simulink model "PEMEC_smlk"  (R2015b)
settings: Solver=VariableStepAuto  SolverMode=SingleTasking  StartTime=0.0  StopTime=1000  MaxStep=1  MinStep=0.0001  RelTol=1e-3
values from neighbouring files (symbols this model uses):
  a = 1 / tau_th + C_cw / C_th * (1 - exp(-UA / C_cw))    [PEMEC_cellstack.m]    (also in PEMEC_data.m = 0.000364)
  A_cell = 0.0170    (= 0.017)    [PEMEC_begin.m]
  alpha_an = 2    [PEMEC_cellstack.m]    (also in PEMEC_data.m)
  alpha_cat = 0.5    [PEMEC_cellstack.m]    (also in PEMEC_data.m)
  b = N_cell * V_ * I * (1 - eta_e) / C_th + T_amb / tau_th +      C_cw * T_cwin / C_th * (1 - exp(-UA / C_cw))    [PEMEC_cellstack.m]    (also in PEMEC_data.m = 2.334)
  C = 0.008    [PEMEC_data.m]
  c_cw = 4.18e03    (= 4180)    [PEMEC_cellstack.m]    (also in PEMEC_data.m)
  C_th = 250e03    (= 250000)    [PEMEC_data.m]
  cH2_me0 = 10.0    (= 10)    [PEMEC_data.m]
  cO2_me0 = 0.10    (= 0.1)    [PEMEC_data.m]
  Deff_an0 = Deff_an_  * 1e04    [PEMEC_data.m]
  Deff_cat0 = Deff_cat_ * 1e04    [PEMEC_data.m]
  DeltaP = (p_an - p_atm) / eta_p    [PEMEC_data.m]
  Dw = 1.28e-10    [PEMEC_cellstack.m]    (also in PEMEC_data.m)
  Epro = 20000    [PEMEC_data.m]
  eta_ACDC = 0.96    [PEMEC_data.m]
  F = 96485    [PEMEC_begin.m]
  f1 = 25000    [PEMEC_data.m]
  f2 = 0.98    [PEMEC_data.m]
  h_cond = 380    [PEMEC_data.m]
  h_conv = 0.1    [PEMEC_data.m]
  K2 = 1 / (2 * A * io_an)    [PEMEC_cellstack.m]    (also in PEMEC_data.m = 1 / (2 * A_cell * io_an))
  K4 = 1 / (2 * A * io_cat)    [PEMEC_cellstack.m]    (also in PEMEC_data.m = 1 / (2 * A_cell * io_cat))
  K_H2 = n_H2r / p_H2out    [PEMEC_data.m]
  K_H2O = n_H2Oout / p_H2Oout    [PEMEC_data.m]
  K_O2 = n_O2r / p_O2out    [PEMEC_data.m]
  K_r = N_cell / (4 * F)    [PEMEC_data.m]
  m_cw = 0.1075    [PEMEC_cellstack.m]    (also in PEMEC_data.m = 0.25)
  M_H2 = 2.01588    [PEMEC_cellstack.m]    (also in PEMEC_data.m)
  M_H2O = 18.01528    [PEMEC_cellstack.m]    (also in PEMEC_data.m)
  M_O2 = 31.9988    [PEMEC_cellstack.m]    (also in PEMEC_data.m)
  N_cell = 200    [PEMEC_begin.m]
  n_H2Omem2 = 1 - Dw / t_mem * (t_cat / Deff_cat + t_an / Deff_an)    [PEMEC_cellstack.m]    (also in PEMEC_data.m = 1 - Dw / t_mem * (t_cat / Deff_cat_ + t_an / Deff_an_))
  n_H2Opg = Kw * A * rho_H2O / (mu_H2O * M_H2O * t_mem) * (p_cat - p_an)    [PEMEC_cellstack.m]    (also in PEMEC_data.m = Kw * A_cell * rho_H2O / (mu_H2O * M_H2O * t_mem)*(p_cat - p_)
  nd = 7    [PEMEC_cellstack.m]    (also in PEMEC_data.m)
  p_an = p_atm * 50    (= 5066250)    [PEMEC_begin.m]
  p_cat = p_atm * 50    (= 5066250)    [PEMEC_begin.m]
  P_gamma = 2.5e03    (= 2500)    [PEMEC_data.m]
  p_H20 = y_H2O * p_an / 101325    [PEMEC_data.m]
  p_H2O0 = y_H2 * p_an / 101325    [PEMEC_data.m]
  p_O20 = y_O2 * p_cat / 101325    [PEMEC_data.m]
  R = 8.314    [PEMEC_begin.m]
  R_th = 0.0817    [PEMEC_data.m]
  Req_el = 180e-06    (= 0.00018)    [PEMEC_data.m]
  rho_H2O = 1000    [PEMEC_cellstack.m]    (also in PEMEC_data.m = 999.7)
  T = 80 + 273.15    (= 353.15)    [PEMEC_begin.m]
  T0 = T_a    [PEMEC_data.m]
  T_a = 25    [PEMEC_begin.m]
  T_amb = 25    [PEMEC_begin.m]    (also in PEMEC_data.m = T_a + 273.15)
  t_an = 0.00020    (= 0.0002)    [PEMEC_data.m]
  t_cat = 0.00020    (= 0.0002)    [PEMEC_data.m]
  T_cwin = 20 + 0    (= 20)    [PEMEC_cellstack.m]    (also in PEMEC_data.m)
  T_des = T - 273.15    [PEMEC_data.m]
  t_mem = 0.00020    (= 0.0002)    [PEMEC_data.m]
  T_ref = 327.15    [PEMEC_begin.m]
  tau_H2 = 2.07    [PEMEC_data.m]
  tau_O2 = 4.14    [PEMEC_data.m]
  tau_p = 0.5    [PEMEC_data.m]
  tau_th = C_th * R_th    [PEMEC_cellstack.m]    (also in PEMEC_data.m = 20425)
  U = polyval(polU, I(1))    [PEMEC_data.m]
  v_H240 = 3.1777e03    (= 3177.7)    [PEMEC_data.m]
  v_H2O = 999.97e03    (= 999970)    [PEMEC_cellstack.m]    (also in PEMEC_data.m = 999700)
  v_O240 = 52.876e03    (= 52876)    [PEMEC_data.m]
  V_tn = 1.48    [PEMEC_cellstack.m]    (also in PEMEC_data.m)
  VS_H2 = 40    [PEMEC_data.m]
  VS_O2 = 20    [PEMEC_data.m]
  y_H2 = 0.005    [PEMEC_begin.m]
  y_O2 = 0.005    [PEMEC_begin.m]
  zeta = 1    [PEMEC_data.m]
undefined symbols (not defined in the file or in its folder): magnitude
settings Model: Creator=gapaolo  LastModifiedBy=gapaolo
settings DataIOCC: SaveFormat=Array
settings OptimizationCC: BlockReduction=off  BooleanDataType=off
settings DebuggingCC: AlgebraicLoopMsg=none  SaveWithParameterizedLinksMsg=none  UnderspecifiedInitializationDetection=Classic  MergeDetectMultiDrivingBlocksExec=none  SignalResolutionControl=TryResolveAllWithWarning
settings HardwareCC: ProdBitPerPointer=32  ProdLargestAtomicFloat=None  ProdIntDivRoundTo=Undefined  ProdEndianess=Unspecified  ProdWordSize=32  ProdHWDeviceType=32-bit Generic  TargetUnknown=on
settings GRTTargetCC: GeneratePreprocessorConditionals=Disable all
settings ConfigComp: CovModelRefEnable=Off  CovSFcnEnable=off

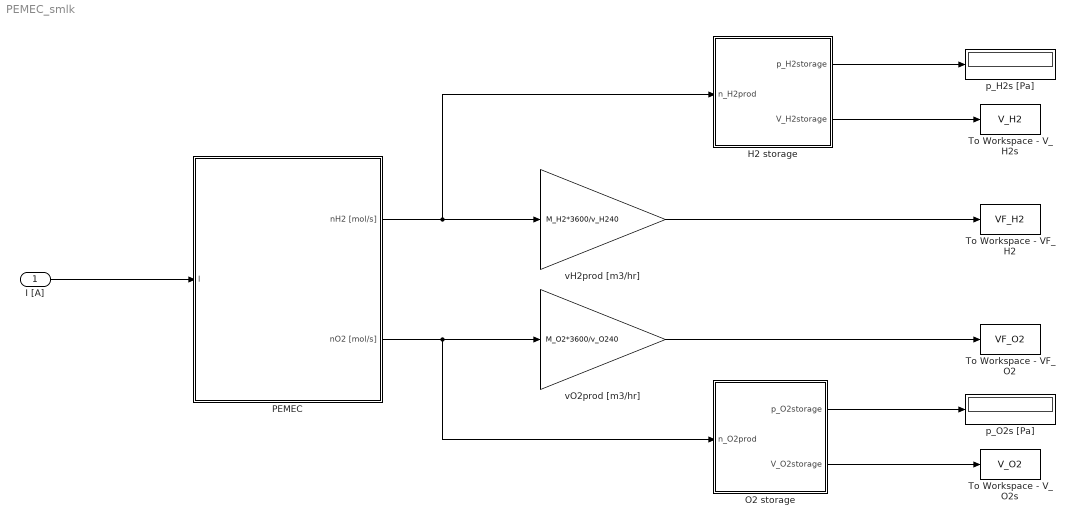
== system PEMEC_smlk ==
  I [A] : Inport
  H2 storage : Subsystem
  O2 storage : Subsystem
  PEMEC : Subsystem
  To Workspace - VF_H2 : ToWorkspace  VariableName=VF_H2  SaveFormat=Timeseries  SampleTime=-1
  To Workspace - VF_O2 : ToWorkspace  VariableName=VF_O2  SaveFormat=Timeseries  SampleTime=-1
  To Workspace - V_H2s : ToWorkspace  VariableName=V_H2  SaveFormat=Timeseries  SampleTime=-1
  To Workspace - V_O2s : ToWorkspace  VariableName=V_O2  SaveFormat=Timeseries  SampleTime=-1
  p_H2s [Pa] : Display
  p_O2s [Pa] : Display
  vH2prod [m3/hr] : Gain  Gain=M_H2*3600/v_H240
  vO2prod [m3/hr] : Gain  Gain=M_O2*3600/v_O240
  wires:
  I [A]/1 -> PEMEC/1(I)
  H2 storage/1(p_H2storage) -> p_H2s [Pa]/1
  PEMEC/2(nO2 [mol/s]) -> O2 storage/1(n_O2prod), vO2prod [m3/hr]/1
  O2 storage/1(p_O2storage) -> p_O2s [Pa]/1
  H2 storage/2(V_H2storage) -> To Workspace - V_H2s/1
  O2 storage/2(V_O2storage) -> To Workspace - V_O2s/1
  vH2prod [m3/hr]/1 -> To Workspace - VF_H2/1
  vO2prod [m3/hr]/1 -> To Workspace - VF_O2/1
  PEMEC/1(nH2 [mol/s]) -> H2 storage/1(n_H2prod), vH2prod [m3/hr]/1

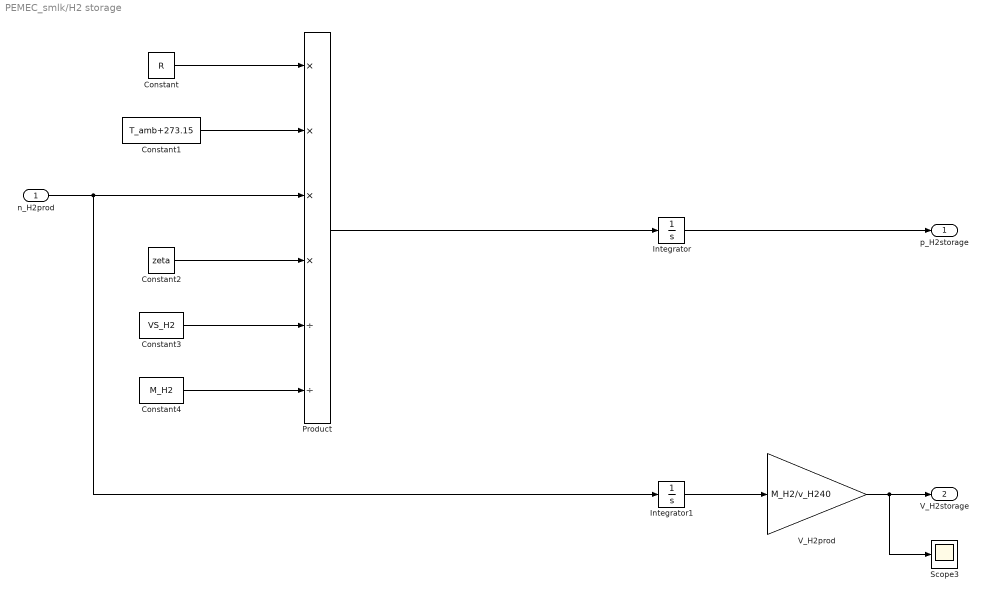
== system PEMEC_smlk/H2 storage ==
  n_H2prod : Inport
  Constant : Constant  Value=R
  Constant1 : Constant  Value=T_amb+273.15
  Constant2 : Constant  Value=zeta
  Constant3 : Constant  Value=VS_H2
  Constant4 : Constant  Value=M_H2
  Integrator : Integrator  InitialCondition=101325
  Integrator1 : Integrator
  Product : Product  Inputs=****//
  Scope3 : Scope
  V_H2prod : Gain  Gain=M_H2/v_H240
  p_H2storage : Outport
  V_H2storage : Outport  Port=2
  wires:
  n_H2prod/1 -> Integrator1/1, Product/3
  Constant/1 -> Product/1
  Constant1/1 -> Product/2
  Constant2/1 -> Product/4
  Constant3/1 -> Product/5
  Constant4/1 -> Product/6
  Product/1 -> Integrator/1
  Integrator/1 -> p_H2storage/1
  Integrator1/1 -> V_H2prod/1
  V_H2prod/1 -> Scope3/1, V_H2storage/1

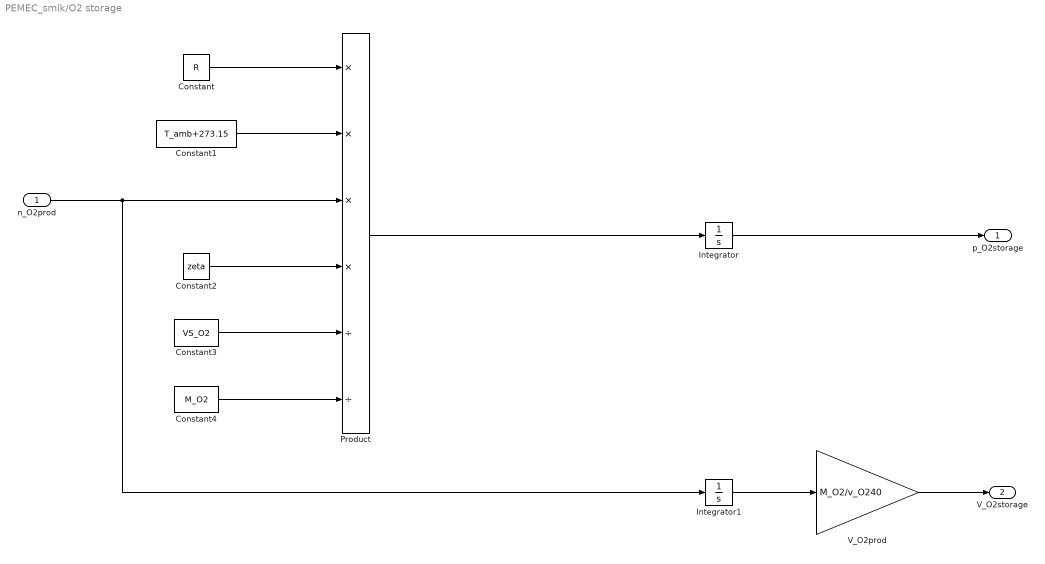
== system PEMEC_smlk/O2 storage ==
  n_O2prod : Inport
  Constant : Constant  Value=R
  Constant1 : Constant  Value=T_amb+273.15
  Constant2 : Constant  Value=zeta
  Constant3 : Constant  Value=VS_O2
  Constant4 : Constant  Value=M_O2
  Integrator : Integrator  InitialCondition=101325
  Integrator1 : Integrator
  Product : Product  Inputs=****//
  V_O2prod : Gain  Gain=M_O2/v_O240
  p_O2storage : Outport
  V_O2storage : Outport  Port=2
  wires:
  n_O2prod/1 -> Integrator1/1, Product/3
  Constant/1 -> Product/1
  Constant1/1 -> Product/2
  Constant2/1 -> Product/4
  Constant3/1 -> Product/5
  Constant4/1 -> Product/6
  Product/1 -> Integrator/1
  Integrator/1 -> p_O2storage/1
  Integrator1/1 -> V_O2prod/1
  V_O2prod/1 -> V_O2storage/1

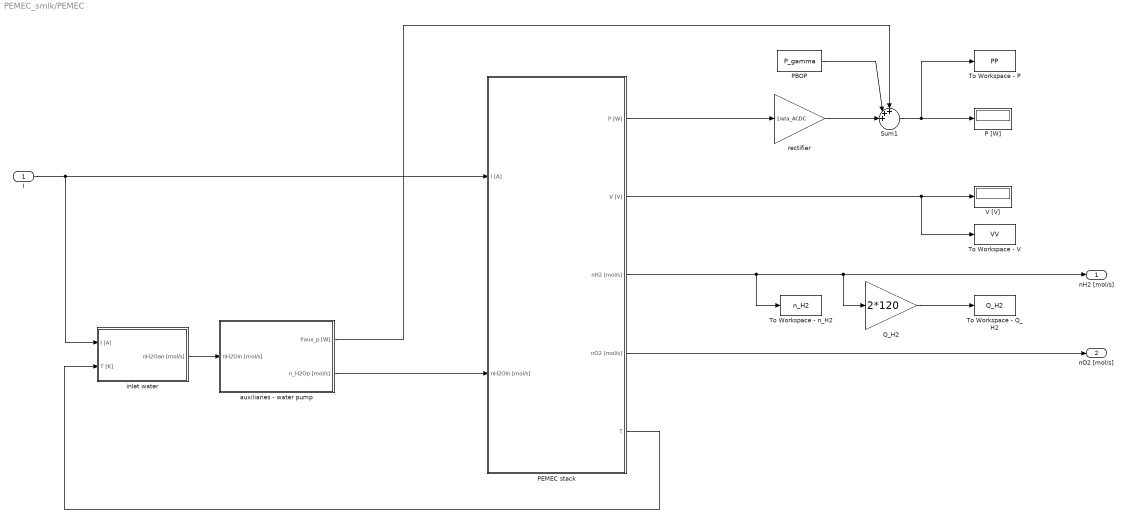
== system PEMEC_smlk/PEMEC ==
  I : Inport
  P [W] : Display
  PBOP : Constant  Value=P_gamma
  PEMEC stack : Subsystem
  Q_H2 : Gain  Gain=2*120
  Sum1 : Sum  Inputs=+++||
  To Workspace - P : ToWorkspace  VariableName=PP  SaveFormat=Timeseries  SampleTime=-1
  To Workspace - Q_H2 : ToWorkspace  VariableName=Q_H2  SaveFormat=Timeseries  SampleTime=-1
  To Workspace - V : ToWorkspace  VariableName=VV  SaveFormat=Timeseries  SampleTime=-1
  To Workspace - n_H2 : ToWorkspace  VariableName=n_H2  SaveFormat=Timeseries  SampleTime=-1
  V [V] : Display
  auxiliaries - water pump : Subsystem
  inlet water : Subsystem
  rectifier : Gain  Gain=1/eta_ACDC
  nH2 [mol/s] : Outport
  nO2 [mol/s] : Outport  Port=2
  wires:
  PEMEC stack/2(V [V]) -> To Workspace - V/1, V [V]/1
  I/1 -> inlet water/1(I [A]), PEMEC stack/1(I [A])
  PEMEC stack/1(P [W]) -> rectifier/1
  inlet water/1("nH2Oan [mol/s] ") -> auxiliaries - water pump/1(nH2Oin [mol/s])
  auxiliaries - water pump/2(n_H2Op [mol/s]) -> PEMEC stack/2(nH2Oin [mol/s])
  rectifier/1 -> Sum1/3
  Sum1/1 -> To Workspace - P/1, P [W]/1
  PBOP/1 -> Sum1/2
  auxiliaries - water pump/1(Paux_p [W]) -> Sum1/1
  PEMEC stack/5(T) -> inlet water/2(T [K])
  PEMEC stack/4(nO2 [mol/s]) -> nO2 [mol/s]/1
  PEMEC stack/3(nH2 [mol/s]) -> Q_H2/1, nH2 [mol/s]/1, To Workspace - n_H2/1
  Q_H2/1 -> To Workspace - Q_H2/1

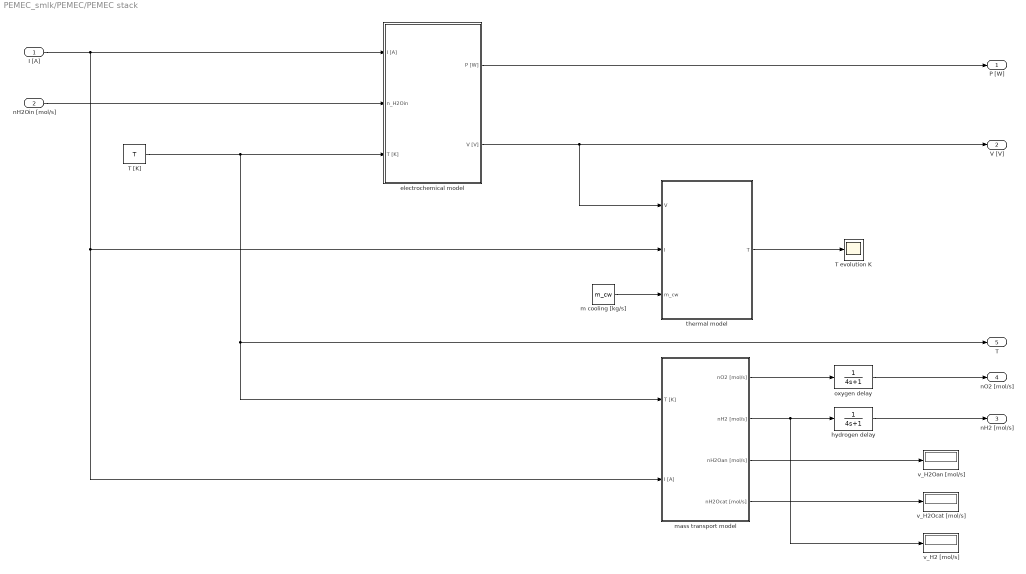
== system PEMEC_smlk/PEMEC/PEMEC stack ==
  I [A] : Inport
  nH2Oin [mol/s] : Inport  Port=2
  T [K] : Constant  Value=T
  T evolution K : Scope
  electrochemical model : Subsystem
  hydrogen delay : TransferFcn  Denominator=[4 1]
  m cooling [kg/s] : Constant  Value=m_cw
  mass transport model : Subsystem
  oxygen delay : TransferFcn  Denominator=[4 1]
  thermal model : Subsystem
  v_H2 [mol/s] : Display
  v_H2Oan [mol/s] : Display
  v_H2Ocat [mol/s] : Display
  P [W] : Outport
  V [V] : Outport  Port=2
  nH2 [mol/s] : Outport  Port=3
  nO2 [mol/s] : Outport  Port=4
  T : Outport  Port=5
  wires:
  m cooling [kg/s]/1 -> thermal model/3(m_cw)
  electrochemical model/2(V [V]) -> V [V]/1, thermal model/1(V)
  thermal model/1(T) -> T evolution K/1
  electrochemical model/1(P [W]) -> P [W]/1
  I [A]/1 -> thermal model/2(I), mass transport model/2(I [A]), electrochemical model/1(I [A])
  nH2Oin [mol/s]/1 -> electrochemical model/2(n_H2Oin)
  T [K]/1 -> T/1, mass transport model/1(T [K]), electrochemical model/3(T [K])
  oxygen delay/1 -> nO2 [mol/s]/1
  hydrogen delay/1 -> nH2 [mol/s]/1
  mass transport model/1(nO2 [mol/s]) -> oxygen delay/1
  mass transport model/2(nH2 [mol/s]) -> v_H2 [mol/s]/1, hydrogen delay/1
  mass transport model/3(nH2Oan [mol/s]) -> v_H2Oan [mol/s]/1
  mass transport model/4(nH2Ocat [mol/s]) -> v_H2Ocat [mol/s]/1

== system PEMEC_smlk/PEMEC/auxiliaries - water pump ==
  nH2Oin [mol/s] : Inport
  Display : Display
  Paux pump : Gain  Gain=DeltaP
  nH2Oin : Gain  Gain=rho_H2O/M_H2O
  pump delay : TransferFcn  Denominator=[tau_p 1]
  vH2in [m3/s] : Gain  Gain=M_H2O/v_H2O
  vH2in [m3/s]1 : Gain  Gain=M_H2O
  Paux_p [W] : Outport
  n_H2Op [mol/s] : Outport  Port=2
  wires:
  vH2in [m3/s]/1 -> pump delay/1
  nH2Oin/1 -> n_H2Op [mol/s]/1
  Paux pump/1 -> Paux_p [W]/1
  nH2Oin [mol/s]/1 -> vH2in [m3/s]1/1, vH2in [m3/s]/1
  pump delay/1 -> nH2Oin/1, Paux pump/1
  vH2in [m3/s]1/1 -> Display/1

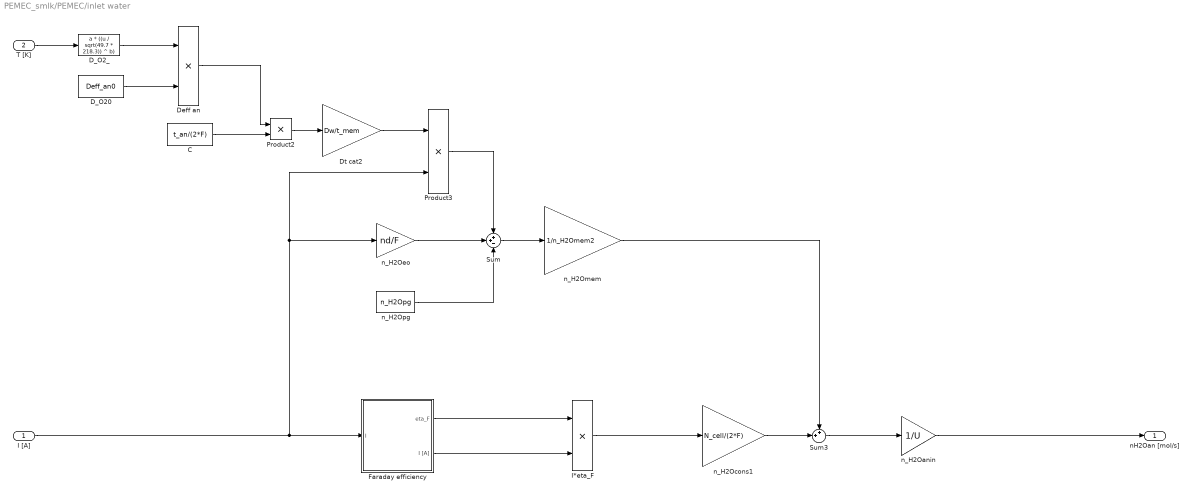
== system PEMEC_smlk/PEMEC/inlet water ==
  I [A] : Inport
  T [K] : Inport  Port=2
  C : Constant  Value=t_an/(2*F)
  D_O20 : Constant  Value=Deff_an0
  D_O2_ : Fcn  Expr=a * ((u / sqrt(49.7 * 218.3)) ^ b)
  Deff an : Product
  Dt cat2 : Gain  Gain=Dw/t_mem
  Faraday efficiency : Subsystem
  I*eta_F : Product
  Product2 : Product
  Product3 : Product
  Sum : Sum  Inputs=++-
  Sum3 : Sum  Inputs=++|
  n_H2Oanin : Gain  Gain=1/U
  n_H2Ocons1 : Gain  Gain=N_cell/(2*F)
  n_H2Oeo : Gain  Gain=nd/F
  n_H2Omem : Gain  Gain=1/n_H2Omem2
  n_H2Opg : Constant  Value=n_H2Opg
  "nH2Oan [mol/s] " : Outport
  wires:
  Faraday efficiency/2(I [A]) -> I*eta_F/2
  Faraday efficiency/1(eta_F) -> I*eta_F/1
  I*eta_F/1 -> n_H2Ocons1/1
  n_H2Opg/1 -> Sum/3
  n_H2Oeo/1 -> Sum/2
  n_H2Ocons1/1 -> Sum3/2
  Sum3/1 -> n_H2Oanin/1
  n_H2Oanin/1 -> "nH2Oan [mol/s] "/1
  Sum/1 -> n_H2Omem/1
  n_H2Omem/1 -> Sum3/1
  I [A]/1 -> Product3/2, n_H2Oeo/1, Faraday efficiency/1(I)
  T [K]/1 -> D_O2_/1
  D_O2_/1 -> Deff an/1
  D_O20/1 -> Deff an/2
  Deff an/1 -> Product2/1
  C/1 -> Product2/2
  Product2/1 -> Dt cat2/1
  Dt cat2/1 -> Product3/1
  Product3/1 -> Sum/1

== system PEMEC_smlk/PEMEC/PEMEC stack/electrochemical model ==
  I [A] : Inport
  n_H2Oin : Inport  Port=2
  T [K] : Inport  Port=3
  Nernst voltage : Subsystem
  P : Product
  "voltage losses " : Subsystem
  P [W] : Outport
  V [V] : Outport  Port=2
  wires:
  I [A]/1 -> Nernst voltage/2(I [A]), "voltage losses "/1(I [A])
  "voltage losses "/1(V) -> P/1, V [V]/1
  P/1 -> P [W]/1
  T [K]/1 -> Nernst voltage/1(T [K]), "voltage losses "/2(T [K])
  "voltage losses "/2(I) -> P/2
  n_H2Oin/1 -> Nernst voltage/3(n_H2Oin)
  Nernst voltage/1(E) -> "voltage losses "/3(E [V])

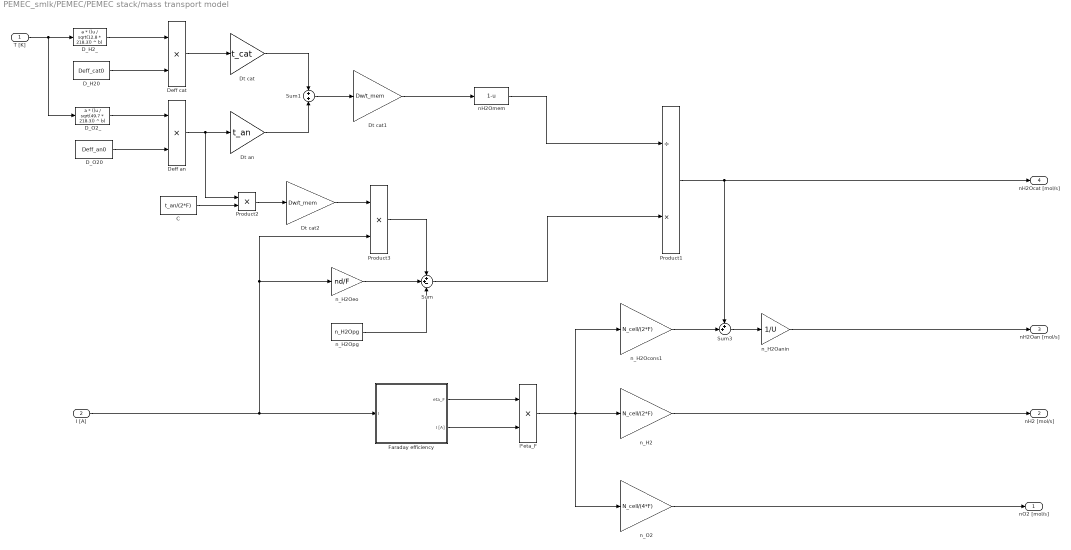
== system PEMEC_smlk/PEMEC/PEMEC stack/mass transport model ==
  T [K] : Inport
  I [A] : Inport  Port=2
  C : Constant  Value=t_an/(2*F)
  D_H20 : Constant  Value=Deff_cat0
  D_H2_ : Fcn  Expr=a * ((u / sqrt(12.8 * 218.3)) ^ b)
  D_O20 : Constant  Value=Deff_an0
  D_O2_ : Fcn  Expr=a * ((u / sqrt(49.7 * 218.3)) ^ b)
  Deff an : Product
  Deff cat : Product
  Dt an : Gain  Gain=t_an
  Dt cat : Gain  Gain=t_cat
  Dt cat1 : Gain  Gain=Dw/t_mem
  Dt cat2 : Gain  Gain=Dw/t_mem
  Faraday efficiency : Subsystem
  I*eta_F : Product
  Product1 : Product  Inputs=/*
  Product2 : Product
  Product3 : Product
  Sum : Sum  Inputs=++-
  Sum1 : Sum  Inputs=+|+
  Sum3 : Sum  Inputs=++|
  nH2Omem : Fcn  Expr=1-u
  n_H2 : Gain  Gain=N_cell/(2*F)
  n_H2Oanin : Gain  Gain=1/U
  n_H2Ocons1 : Gain  Gain=N_cell/(2*F)
  n_H2Oeo : Gain  Gain=nd/F
  n_H2Opg : Constant  Value=n_H2Opg
  n_O2 : Gain  Gain=N_cell/(4*F)
  nO2 [mol/s] : Outport
  nH2 [mol/s] : Outport  Port=2
  nH2Oan [mol/s] : Outport  Port=3
  nH2Ocat [mol/s] : Outport  Port=4
  wires:
  Faraday efficiency/2(I [A]) -> I*eta_F/2
  Faraday efficiency/1(eta_F) -> I*eta_F/1
  n_H2/1 -> nH2 [mol/s]/1
  n_O2/1 -> nO2 [mol/s]/1
  I [A]/1 -> Faraday efficiency/1(I), Product3/2, n_H2Oeo/1
  I*eta_F/1 -> n_H2Ocons1/1, n_H2/1, n_O2/1
  n_H2Opg/1 -> Sum/3
  n_H2Oeo/1 -> Sum/2
  n_H2Ocons1/1 -> Sum3/2
  Sum3/1 -> n_H2Oanin/1
  n_H2Oanin/1 -> nH2Oan [mol/s]/1
  T [K]/1 -> D_H2_/1, D_O2_/1
  D_H2_/1 -> Deff cat/1
  D_O2_/1 -> Deff an/1
  D_H20/1 -> Deff cat/2
  D_O20/1 -> Deff an/2
  Deff cat/1 -> Dt cat/1
  Deff an/1 -> Product2/1, Dt an/1
  Dt cat/1 -> Sum1/1
  Dt an/1 -> Sum1/2
  Sum1/1 -> Dt cat1/1
  Dt cat1/1 -> nH2Omem/1
  Sum/1 -> Product1/2
  nH2Omem/1 -> Product1/1
  Product1/1 -> Sum3/1, nH2Ocat [mol/s]/1
  C/1 -> Product2/2
  Product2/1 -> Dt cat2/1
  Dt cat2/1 -> Product3/1
  Product3/1 -> Sum/1

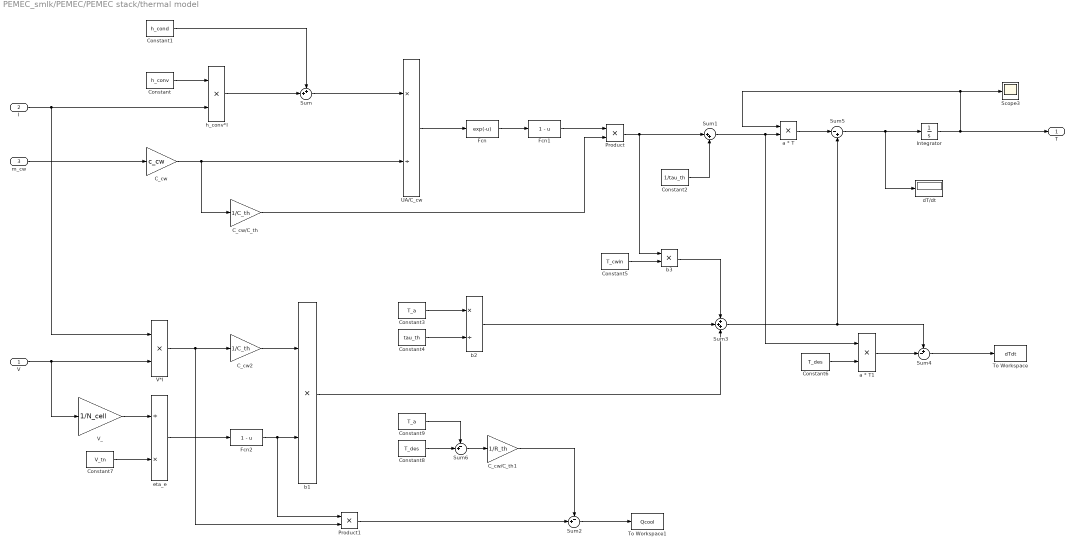
== system PEMEC_smlk/PEMEC/PEMEC stack/thermal model ==
  V : Inport
  I : Inport  Port=2
  m_cw : Inport  Port=3
  C_cw : Gain  Gain=c_cw
  C_cw/C_th : Gain  Gain=1/C_th
  C_cw/C_th1 : Gain  Gain=1/R_th
  C_cw2 : Gain  Gain=1/C_th
  Constant : Constant  Value=h_conv
  Constant1 : Constant  Value=h_cond
  Constant2 : Constant  Value=1/tau_th
  Constant3 : Constant  Value=T_a
  Constant4 : Constant  Value=tau_th
  Constant5 : Constant  Value=T_cwin
  Constant6 : Constant  Value=T_des
  Constant7 : Constant  Value=V_tn
  Constant8 : Constant  Value=T_des
  Constant9 : Constant  Value=T_a
  Fcn : Fcn  Expr=exp(-u)
  Fcn1 : Fcn  Expr=1 - u
  Fcn2 : Fcn  Expr=1 - u
  Integrator : Integrator  InitialCondition=T0
  Product : Product
  Product1 : Product
  Scope3 : Scope
  Sum : Sum  Inputs=++|
  Sum1 : Sum  Inputs=|++
  Sum2 : Sum  Inputs=-+|
  Sum3 : Sum  Inputs=+++
  Sum4 : Sum  Inputs=+-|
  Sum5 : Sum  Inputs=|-+
  Sum6 : Sum  Inputs=-+|
  To Workspace : ToWorkspace  VariableName=dTdt  SaveFormat=Timeseries  SampleTime=-1
  To Workspace1 : ToWorkspace  VariableName=Qcool  SaveFormat=Timeseries  SampleTime=-1
  UA/C_cw : Product  Inputs=*/
  V*I : Product
  V_ : Gain  Gain=1/N_cell
  a * T : Product
  a * T1 : Product
  b1 : Product
  b2 : Product  Inputs=*/
  b3 : Product
  dT/dt : Display
  eta_e : Product  Inputs=/*
  h_conv*I : Product
  T : Outport
  wires:
  I/1 -> V*I/1, h_conv*I/2
  Constant/1 -> h_conv*I/1
  h_conv*I/1 -> Sum/2
  Constant1/1 -> Sum/1
  Sum/1 -> UA/C_cw/1
  m_cw/1 -> C_cw/1
  UA/C_cw/1 -> Fcn/1
  Fcn/1 -> Fcn1/1
  C_cw/1 -> UA/C_cw/2, C_cw/C_th/1
  Fcn1/1 -> Product/1
  C_cw/C_th/1 -> Product/2
  Product/1 -> b3/1, Sum1/1
  Constant2/1 -> Sum1/2
  C_cw2/1 -> b1/1
  Constant3/1 -> b2/1
  Constant4/1 -> b2/2
  Constant5/1 -> b3/2
  b3/1 -> Sum3/1
  b2/1 -> Sum3/2
  V_/1 -> eta_e/1
  Constant7/1 -> eta_e/2
  eta_e/1 -> Fcn2/1
  Sum5/1 -> dT/dt/1, Integrator/1
  a * T/1 -> Sum5/1
  Sum1/1 -> a * T1/1, a * T/2
  Integrator/1 -> a * T/1, Scope3/1, T/1
  b1/1 -> Sum3/3
  Sum3/1 -> Sum4/1, Sum5/2
  Constant6/1 -> a * T1/2
  Sum4/1 -> To Workspace/1
  a * T1/1 -> Sum4/2
  Product1/1 -> Sum2/2
  Constant8/1 -> Sum6/2
  Constant9/1 -> Sum6/1
  Sum6/1 -> C_cw/C_th1/1
  C_cw/C_th1/1 -> Sum2/1
  Sum2/1 -> To Workspace1/1
  V*I/1 -> Product1/2, C_cw2/1
  Fcn2/1 -> Product1/1, b1/2
  V/1 -> V*I/2, V_/1

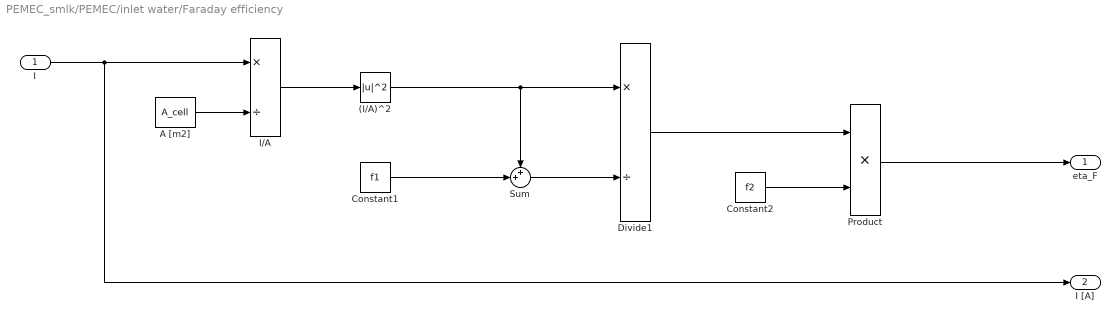
== system PEMEC_smlk/PEMEC/inlet water/Faraday efficiency ==
  I : Inport
  (I/A)^2 : Math  Operator=magnitude^2  SaturateOnIntegerOverflow=on
  A [m2] : Constant  Value=A_cell
  Constant1 : Constant  Value=f1
  Constant2 : Constant  Value=f2
  Divide1 : Product  Inputs=*/
  I/A : Product  Inputs=*/
  Product : Product
  Sum : Sum  Inputs=++|
  eta_F : Outport
  I [A] : Outport  Port=2
  wires:
  A [m2]/1 -> I/A/2
  I/1 -> I [A]/1, I/A/1
  I/A/1 -> (I/A)^2/1
  (I/A)^2/1 -> Sum/1, Divide1/1
  Constant1/1 -> Sum/2
  Sum/1 -> Divide1/2
  Divide1/1 -> Product/1
  Constant2/1 -> Product/2
  Product/1 -> eta_F/1

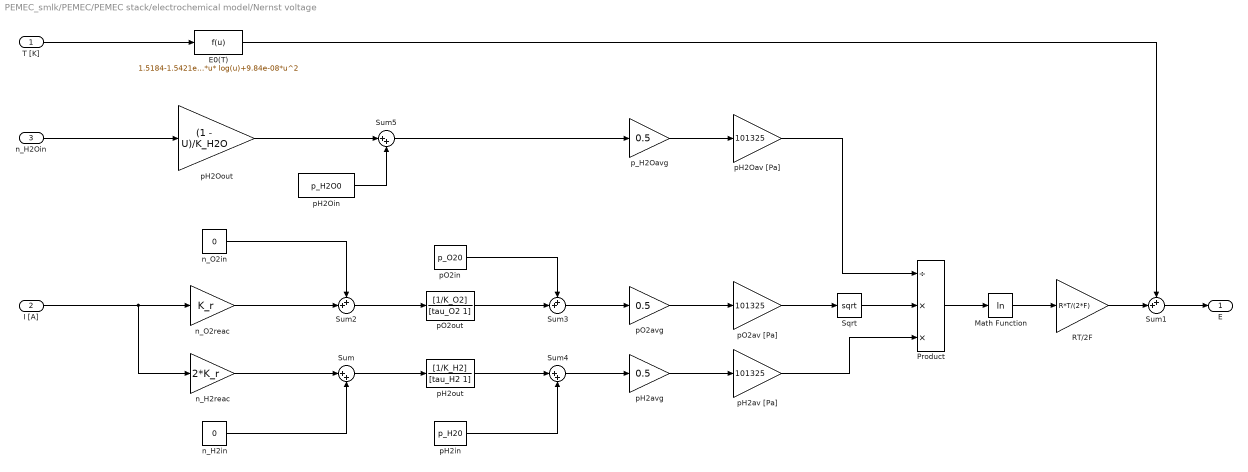
== system PEMEC_smlk/PEMEC/PEMEC stack/electrochemical model/Nernst voltage ==
  T [K] : Inport
  I [A] : Inport  Port=2
  n_H2Oin : Inport  Port=3
  E0(T) : Fcn  Expr=1.5184-1.5421e-03*u+9.523e-05*u* log(u)+9.84e-08*u^2
  Math Function : Math  Operator=log  SaturateOnIntegerOverflow=on
  Product : Product  Inputs=/**
  RT/2F : Gain  Gain=R*T/(2*F)
  Sqrt : Sqrt  SaturateOnIntegerOverflow=on
  Sum : Sum  Inputs=|++
  Sum1 : Sum  Inputs=++|
  Sum2 : Sum  Inputs=++|
  Sum3 : Sum  Inputs=++|
  Sum4 : Sum  Inputs=|++
  Sum5 : Sum  Inputs=|++
  n_H2in : Constant  Value=0
  n_H2reac : Gain  Gain=2*K_r
  n_O2in : Constant  Value=0
  n_O2reac : Gain  Gain=K_r
  pH2Oav [Pa] : Gain  Gain=101325
  pH2Oin : Constant  Value=p_H2O0
  pH2Oout : Gain  Gain=(1 - U)/K_H2O
  pH2av [Pa] : Gain  Gain=101325
  pH2avg : Gain  Gain=0.5
  pH2in : Constant  Value=p_H20
  pH2out : TransferFcn  Numerator=[1/K_H2]  Denominator=[tau_H2 1]  ContinuousStateAttributes='p_H2'
  pO2av [Pa] : Gain  Gain=101325
  pO2avg : Gain  Gain=0.5
  pO2in : Constant  Value=p_O20
  pO2out : TransferFcn  Numerator=[1/K_O2]  Denominator=[tau_O2 1]  ContinuousStateAttributes='p_O2'
  p_H2Oavg : Gain  Gain=0.5
  E : Outport
  wires:
  I [A]/1 -> n_O2reac/1, n_H2reac/1
  n_H2reac/1 -> Sum/1
  Sum/1 -> pH2out/1
  Sum2/1 -> pO2out/1
  RT/2F/1 -> Sum1/2
  E0(T)/1 -> Sum1/1
  pH2out/1 -> Sum4/1
  pO2out/1 -> Sum3/2
  pH2in/1 -> Sum4/2
  pO2in/1 -> Sum3/1
  Sum1/1 -> E/1
  n_O2reac/1 -> Sum2/2
  n_O2in/1 -> Sum2/1
  n_H2in/1 -> Sum/2
  Sqrt/1 -> Product/2
  Product/1 -> Math Function/1
  Math Function/1 -> RT/2F/1
  pO2av [Pa]/1 -> Sqrt/1
  pH2av [Pa]/1 -> Product/3
  Sum5/1 -> p_H2Oavg/1
  n_H2Oin/1 -> pH2Oout/1
  pH2Oin/1 -> Sum5/2
  pH2Oout/1 -> Sum5/1
  p_H2Oavg/1 -> pH2Oav [Pa]/1
  Sum3/1 -> pO2avg/1
  Sum4/1 -> pH2avg/1
  T [K]/1 -> E0(T)/1
  pH2Oav [Pa]/1 -> Product/1
  pO2avg/1 -> pO2av [Pa]/1
  pH2avg/1 -> pH2av [Pa]/1

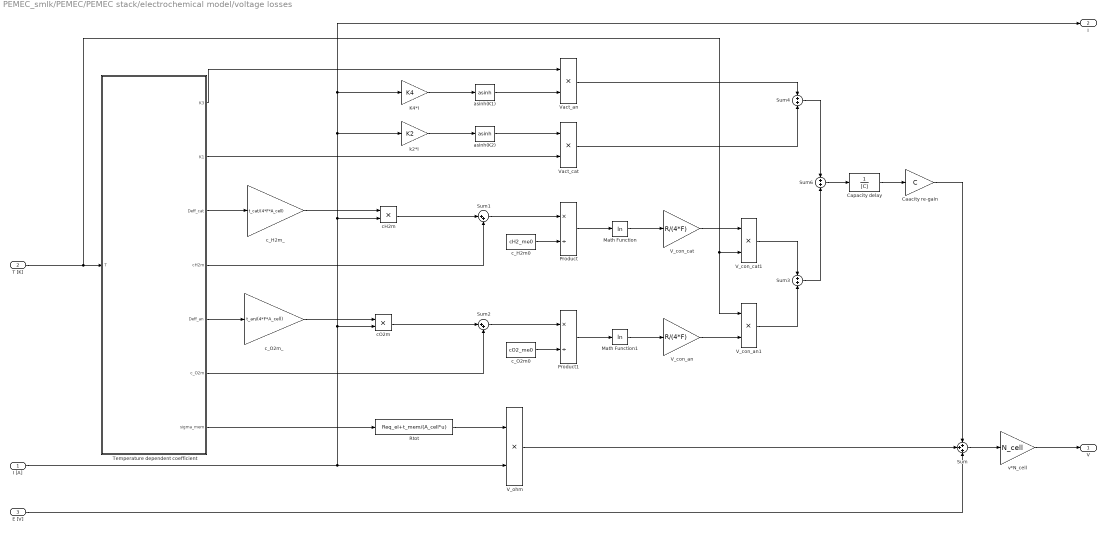
== system PEMEC_smlk/PEMEC/PEMEC stack/electrochemical model/voltage losses  ==
  I [A] : Inport
  T [K] : Inport  Port=2
  E [V] : Inport  Port=3
  Caacity re-gain : Gain  Gain=C
  Capacity delay : TransferFcn  Denominator=[C]
  K4*I : Gain  Gain=K4
  Math Function : Math  Operator=log  SaturateOnIntegerOverflow=on
  Math Function1 : Math  Operator=log  SaturateOnIntegerOverflow=on
  Product : Product  Inputs=*/
  Product1 : Product  Inputs=*/
  Rtot : Fcn  Expr=Req_el+t_mem/(A_cell*u)
  Sum : Sum  Inputs=+++
  Sum1 : Sum  Inputs=|++
  Sum2 : Sum  Inputs=|++
  Sum3 : Sum  Inputs=+|+
  Sum4 : Sum  Inputs=+|+
  Sum6 : Sum  Inputs=+|+
  Temperature dependent coefficient : Subsystem
  V_con_an : Gain  Gain=R/(4*F)
  V_con_an1 : Product
  V_con_cat : Gain  Gain=R/(4*F)
  V_con_cat1 : Product
  V_ohm : Product
  Vact_an : Product
  Vact_cat : Product
  asinh(K1) : Trigonometry  Operator=asinh
  asinh(K2) : Trigonometry  Operator=asinh
  cH2m : Product
  cO2m : Product
  c_H2m0 : Constant  Value=cH2_me0
  c_H2m_ : Gain  Gain=t_cat/(4*F*A_cell)
  c_O2m0 : Constant  Value=cO2_me0
  c_O2m_ : Gain  Gain=t_an/(4*F*A_cell)
  k2*I : Gain  Gain=K2
  v*N_cell : Gain  Gain=N_cell
  V : Outport
  I : Outport  Port=2
  wires:
  I [A]/1 -> cO2m/2, cH2m/2, I/1, K4*I/1, k2*I/1, V_ohm/2
  Sum/1 -> v*N_cell/1
  cH2m/1 -> Sum1/1
  Temperature dependent coefficient/4(cH2m) -> Sum1/2
  Temperature dependent coefficient/6(c_O2m) -> Sum2/2
  cO2m/1 -> Sum2/1
  c_H2m0/1 -> Product/2
  Sum1/1 -> Product/1
  Sum2/1 -> Product1/1
  c_O2m0/1 -> Product1/2
  Product/1 -> Math Function/1
  Product1/1 -> Math Function1/1
  Math Function/1 -> V_con_cat/1
  Math Function1/1 -> V_con_an/1
  k2*I/1 -> asinh(K2)/1
  K4*I/1 -> asinh(K1)/1
  asinh(K2)/1 -> Vact_cat/1
  asinh(K1)/1 -> Vact_an/2
  Vact_cat/1 -> Sum4/2
  Vact_an/1 -> Sum4/1
  Sum4/1 -> Sum6/1
  Temperature dependent coefficient/1(K3) -> Vact_an/1
  Temperature dependent coefficient/2(K1) -> Vact_cat/2
  V_con_cat1/1 -> Sum3/1
  V_con_cat/1 -> V_con_cat1/1
  V_con_an/1 -> V_con_an1/2
  V_con_an1/1 -> Sum3/2
  Temperature dependent coefficient/7(sigma_mem) -> Rtot/1
  Rtot/1 -> V_ohm/1
  V_ohm/1 -> Sum/2
  Capacity delay/1 -> Caacity re-gain/1
  Sum3/1 -> Sum6/2
  Sum6/1 -> Capacity delay/1
  Caacity re-gain/1 -> Sum/1
  E [V]/1 -> Sum/3
  v*N_cell/1 -> V/1
  T [K]/1 -> V_con_an1/1, V_con_cat1/2, Temperature dependent coefficient/1(T)
  Temperature dependent coefficient/5(Deff_an) -> c_O2m_/1
  Temperature dependent coefficient/3(Deff_cat) -> c_H2m_/1
  c_O2m_/1 -> cO2m/1
  c_H2m_/1 -> cH2m/1

== system PEMEC_smlk/PEMEC/PEMEC stack/mass transport model/Faraday efficiency ==
  I : Inport
  (I/A)^2 : Math  Operator=magnitude^2  SaturateOnIntegerOverflow=on
  A [m2] : Constant  Value=A_cell
  Constant1 : Constant  Value=f1
  Constant2 : Constant  Value=f2
  Divide1 : Product  Inputs=*/
  I/A : Product  Inputs=*/
  Product : Product
  Sum : Sum  Inputs=++|
  eta_F : Outport
  I [A] : Outport  Port=2
  wires:
  A [m2]/1 -> I/A/2
  I/1 -> I [A]/1, I/A/1
  I/A/1 -> (I/A)^2/1
  (I/A)^2/1 -> Sum/1, Divide1/1
  Constant1/1 -> Sum/2
  Sum/1 -> Divide1/2
  Divide1/1 -> Product/1
  Constant2/1 -> Product/2
  Product/1 -> eta_F/1

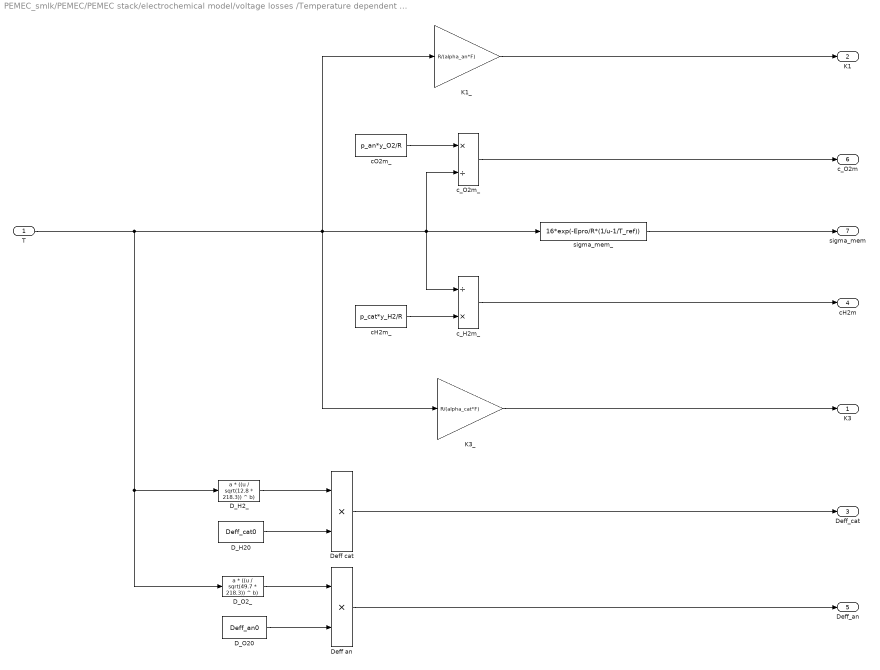
== system PEMEC_smlk/PEMEC/PEMEC stack/electrochemical model/voltage losses /Temperature dependent coefficient ==
  T : Inport
  D_H20 : Constant  Value=Deff_cat0
  D_H2_ : Fcn  Expr=a * ((u / sqrt(12.8 * 218.3)) ^ b)
  D_O20 : Constant  Value=Deff_an0
  D_O2_ : Fcn  Expr=a * ((u / sqrt(49.7 * 218.3)) ^ b)
  Deff an : Product
  Deff cat : Product
  K1_ : Gain  Gain=R/(alpha_an*F)
  K3_ : Gain  Gain=R/(alpha_cat*F)
  cH2m_ : Constant  Value=p_cat*y_H2/R
  cO2m_ : Constant  Value=p_an*y_O2/R
  c_H2m_ : Product  Inputs=/*
  c_O2m_ : Product  Inputs=*/
  sigma_mem_ : Fcn  Expr=16*exp(-Epro/R*(1/u-1/T_ref))
  K3 : Outport
  K1 : Outport  Port=2
  Deff_cat : Outport  Port=3
  cH2m : Outport  Port=4
  Deff_an : Outport  Port=5
  c_O2m : Outport  Port=6
  sigma_mem : Outport  Port=7
  wires:
  cO2m_/1 -> c_O2m_/1
  cH2m_/1 -> c_H2m_/2
  T/1 -> D_O2_/1, D_H2_/1, K3_/1, K1_/1, sigma_mem_/1, c_H2m_/1, c_O2m_/2
  c_H2m_/1 -> cH2m/1
  c_O2m_/1 -> c_O2m/1
  sigma_mem_/1 -> sigma_mem/1
  K3_/1 -> K3/1
  K1_/1 -> K1/1
  D_H2_/1 -> Deff cat/1
  D_O2_/1 -> Deff an/1
  D_H20/1 -> Deff cat/2
  D_O20/1 -> Deff an/2
  Deff cat/1 -> Deff_cat/1
  Deff an/1 -> Deff_an/1
